simulink subsystem "brakelight"  (R2022b)
settings: Solver=VariableStepAuto  StartTime=0.0  StopTime=10.0  RelTol=1e-3
libraries: brake_lib x1, Raptor_lib x1
settings Model: Creator=serga  LastModifiedBy=serga

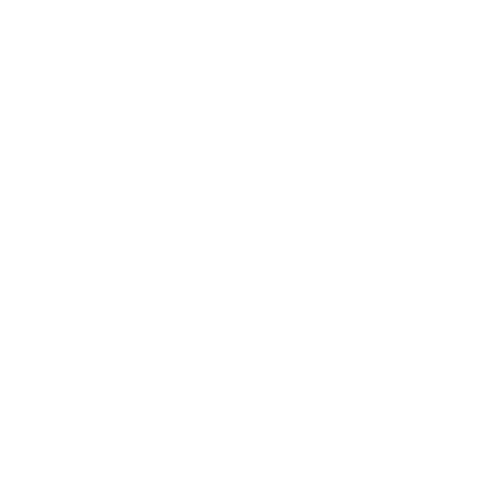
[thumbnail: Simulink's stored preview of the top-level diagram]
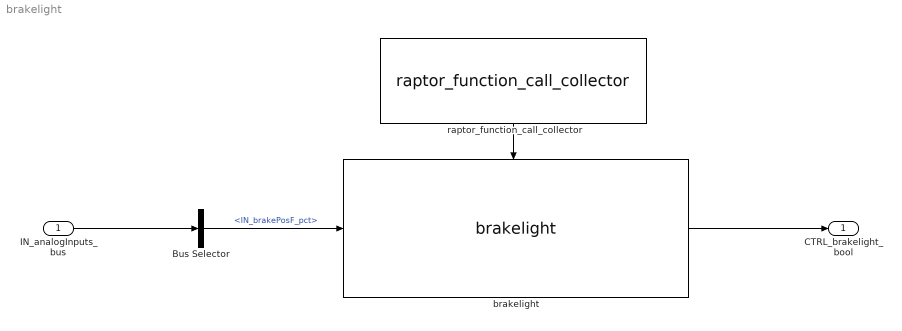
== system brakelight ==
  IN_analogInputs_bus : Inport
  Bus Selector : BusSelector  OutputSignals=IN_brake_bus.IN_brakeF_bus.IN_brakePosF_pct
  brakelight : brake_lib/brakelight  SystemSampleTime=-1  VariantActivationTime=update diagram  Latency=0  AutoFrameSizeCalculation=off
  raptor_function_call_collector : Raptor_lib/Triggers/raptor_function_call_collector  count=5
      settings: SourceProductName=Raptor
  CTRL_brakelight_bool : Outport
  wires:
  IN_analogInputs_bus/1 -> Bus Selector/1
  Bus Selector/1 -> brakelight/1  "<IN_brakePosF_pct>"
  raptor_function_call_collector/1 -> brakelight/Trigger
  brakelight/1 -> CTRL_brakelight_bool/1
